simulink model "control_system_2022b"  (R2022b)
settings: Solver=VariableStepAuto  StartTime=0.0  StopTime=10.0  RelTol=1e-3
model workspace (MAT data in the model file):
  b_w = Simulink.Parameter
  b_w.Value = 150
  b_w.DataType = 'auto'
  b_w.Complexity = 'real'
  b_w.Dimensions = [1 1]
  v = Simulink.Parameter
  v.Value = 1000
  v.DataType = 'auto'
  v.Complexity = 'real'
  v.Dimensions = [1 1]
libraries: slpidlib x3
settings Model: Creator=gabrielle  LastModifiedBy=22546723@sun.ac.za
settings OptimizationCC: ReuseModelBlockBuffer=on

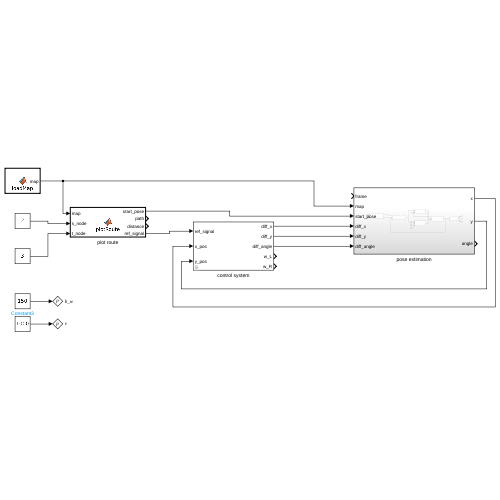
[thumbnail: Simulink's stored preview of the top-level diagram]
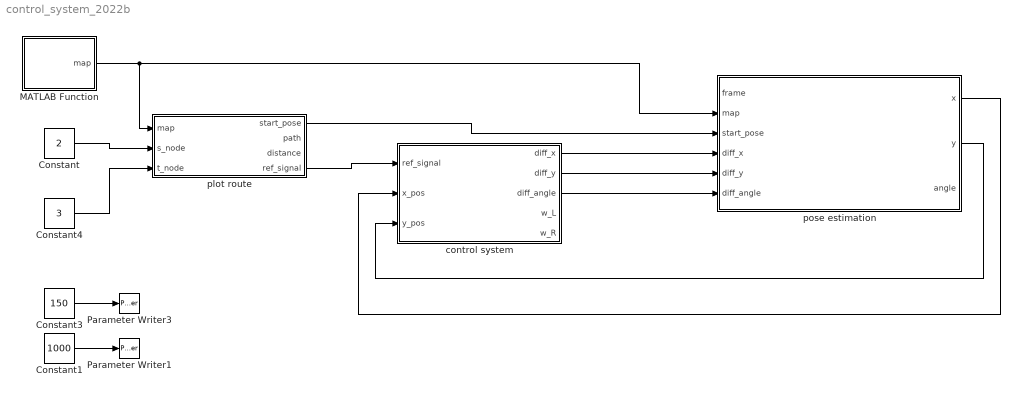
== system control_system_2022b ==
  Constant : Constant  Value=2
  Constant1 : Constant  Value=1000
  Constant3 : Constant  Value=150
  Constant4 : Constant  Value=3
  MATLAB Function : MATLAB Function  TreatAsAtomicUnit=on
  Parameter Writer1 : ParameterWriter  AccessWorkspaceVariable=on  WorkspaceVariableName=v
  Parameter Writer3 : ParameterWriter  AccessWorkspaceVariable=on  WorkspaceVariableName=b_w
  control system : Subsystem  mask{b_w=b_w, V=v}
      mask prompts: b_w "Distance between drive whels (mm)"; V "Base wheel speed (mm/s)"
  plot route : MATLAB Function  TreatAsAtomicUnit=on
  pose estimation : Subsystem
  wires:
  Constant3/1 -> Parameter Writer3/1
  Constant1/1 -> Parameter Writer1/1
  plot route/4(ref_signal) -> control system/1(ref_signal)
  control system/1(diff_x) -> pose estimation/4(diff_x)
  control system/2(diff_y) -> pose estimation/5(diff_y)
  control system/3(diff_angle) -> pose estimation/6(diff_angle)
  pose estimation/1(x) -> control system/2(x_pos)
  pose estimation/2(y) -> control system/3(y_pos)
  MATLAB Function/1(map) -> plot route/1(map), pose estimation/2(map)
  Constant/1 -> plot route/2(s_node)
  Constant4/1 -> plot route/3(t_node)
  plot route/1(start_pose) -> pose estimation/3(start_pose)

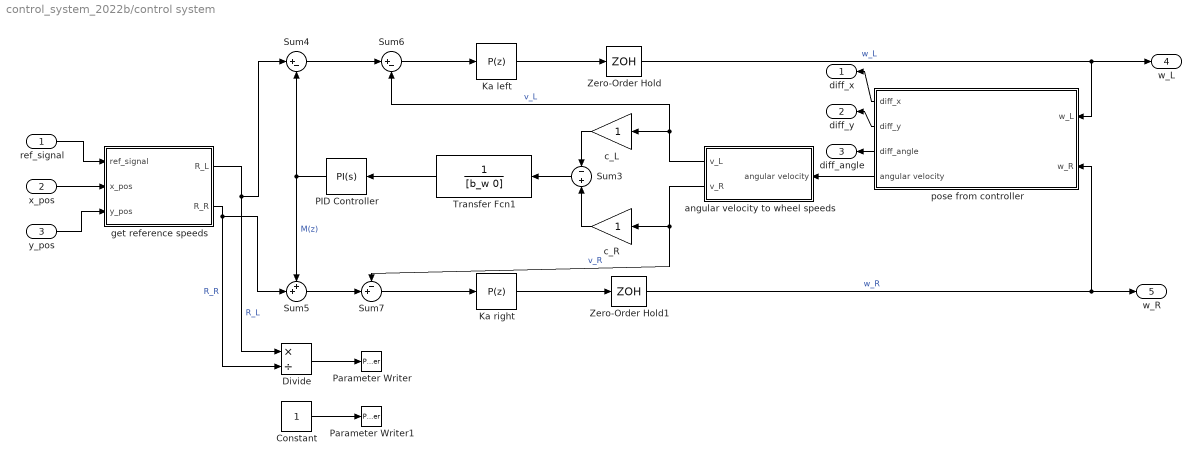
== system control_system_2022b/control system ==
  ref_signal : Inport
  x_pos : Inport  Port=2
  y_pos : Inport  Port=3
  Constant : Constant
  Divide : Product  Inputs=*/
  Ka left : slpidlib/PID Controller  Controller=P  Form=Parallel  TimeDomain=Discrete-time  UseExternalTs=off  SampleTime=-1  IntegratorMethod=Forward Euler  FilterMethod=Forward Euler  ControllerParametersSource=internal  P=1  I=1  UseKiTs=off  D=0  N=100  UseFilter=on  TunerSelectOption=Transfer Function Based (PID Tuner App)  InitialConditionSource=internal  InitialConditionForIntegrator=0  InitialConditionForFilter=0  DifferentiatorICPrevScaledInput=0  ExternalReset=none  TrackingMode=off  Kt=1  LimitOutput=off  SatLimitsSource=internal  UpperSaturationLimit=inf  LowerSaturationLimit=-inf  LinearizeAsGain=off  AntiWindupMode=none  Kb=1  LimitIntegrator=off  UpperIntegratorSaturationLimit=inf  LowerIntegratorSaturationLimit=-inf  POutMin=[]  POutMax=[]  IOutMin=[]  IOutMax=[]  DOutMin=[]  DOutMax=[]  NOutMin=[]  NOutMax=[]  SumOutMin=[]  SumOutMax=[]  SaturationOutMin=[]  SaturationOutMax=[]  PParamMin=[]  PParamMax=[]  IParamMin=[]  IParamMax=[]  DParamMin=[]  DParamMax=[]  NParamMin=[]  NParamMax=[]  KbParamMin=[]  KbParamMax=[]  KtParamMin=[]  KtParamMax=[]  KbOutMin=[]  KbOutMax=[]  KtOutMin=[]  KtOutMax=[]  IntegratorOutMin=[]  IntegratorOutMax=[]  FilterOutMin=[]  FilterOutMax=[]  SumI1OutMin=[]  SumI1OutMax=[]  SumI2OutMin=[]  SumI2OutMax=[]  SumI3OutMin=[]  SumI3OutMax=[]  SumI4OutMin=[]  SumI4OutMax=[]  SumDOutMin=[]  SumDOutMax=[]  DifferentiatorOutMin=[]  DifferentiatorOutMax=[]  FilterDiffOutCoefMin=[]  FilterDiffOutCoefMax=[]  ReciprocalOutMin=[]  ReciprocalOutMax=[]  SumDenOutMin=[]  SumDenOutMax=[]  SumNumOutMin=[]  SumNumOutMax=[]  DivideOutMin=[]  DivideOutMax=[]  UdiffTsProdOutMin=[]  UdiffTsProdOutMax=[]  NTsProdOutMin=[]  NTsProdOutMax=[]  UintegralTsProdOutMin=[]  UintegralTsProdOutMax=[]  UngainTsProdOutMin=[]  UngainTsProdOutMax=[]  ClampingZeroOutDataTypeStr=Inherit: Inherit via back propagation  ClampingZeroOutMin=[]  ClampingZeroOutMax=[]  FilterDenConstantOutDataTypeStr=Inherit: Inherit via back propagation  FilterDenConstantOutMin=[]  FilterDenConstantOutMax=[]  PCopyOutDataTypeStr=Inherit: Inherit via back propagation  PCopyOutMin=[]  PCopyOutMax=[]  NCopyOutDataTypeStr=Inherit: Inherit via back propagation  NCopyOutMin=[]  NCopyOutMax=[]  IntegratorContinuousStateAttributes=''  IntegratorStateMustResolveToSignalObject=off  IntegratorRTWStateStorageClass=Auto  FilterContinuousStateAttributes=''  FilterStateMustResolveToSignalObject=off  FilterRTWStateStorageClass=Auto  ParallelPVariant=InternalParameters  IdealPVariant=Disabled  IVariant=Disabled  DVariant=Disabled  IntegratorVariant=Disabled  SatVariant=Disabled  AWVariant=Disabled  PCopyVariant=Disabled  TRVariant=Disabled  FdbkBlocksVariant=Forward  IdealPFdbkVariant=Disabled  SatFdbkVariant=Disabled  DerivativeFilterVariant=Disabled  NVariant=Disabled  NCopyVariant=Disabled_SignalSpec  FilterICVariant=Disabled  IntegratorICVariant=Disabled  ExternalResetVariant=Disabled  TRSumVariant=Passthrough  SumFdbkVariant=Disabled  SumVariant=Passthrough_P  TsampFilterVariant=InternalTs  TsampNgainVariant=Passthrough  TsampIntegralVariant=Disabled_SignalSpec  ExternalSaturationOutDataTypeStr=Inherit: Same as second input
      settings: LibrarySourceBlock=simulink/Discrete/Discrete PID Controller
  Ka right : slpidlib/PID Controller  Controller=P  Form=Parallel  TimeDomain=Discrete-time  UseExternalTs=off  SampleTime=-1  IntegratorMethod=Forward Euler  FilterMethod=Forward Euler  ControllerParametersSource=internal  P=1  I=1  UseKiTs=off  D=0  N=100  UseFilter=on  TunerSelectOption=Transfer Function Based (PID Tuner App)  InitialConditionSource=internal  InitialConditionForIntegrator=0  InitialConditionForFilter=0  DifferentiatorICPrevScaledInput=0  ExternalReset=none  TrackingMode=off  Kt=1  LimitOutput=off  SatLimitsSource=internal  UpperSaturationLimit=inf  LowerSaturationLimit=-inf  LinearizeAsGain=off  AntiWindupMode=none  Kb=1  LimitIntegrator=off  UpperIntegratorSaturationLimit=inf  LowerIntegratorSaturationLimit=-inf  POutMin=[]  POutMax=[]  IOutMin=[]  IOutMax=[]  DOutMin=[]  DOutMax=[]  NOutMin=[]  NOutMax=[]  SumOutMin=[]  SumOutMax=[]  SaturationOutMin=[]  SaturationOutMax=[]  PParamMin=[]  PParamMax=[]  IParamMin=[]  IParamMax=[]  DParamMin=[]  DParamMax=[]  NParamMin=[]  NParamMax=[]  KbParamMin=[]  KbParamMax=[]  KtParamMin=[]  KtParamMax=[]  KbOutMin=[]  KbOutMax=[]  KtOutMin=[]  KtOutMax=[]  IntegratorOutMin=[]  IntegratorOutMax=[]  FilterOutMin=[]  FilterOutMax=[]  SumI1OutMin=[]  SumI1OutMax=[]  SumI2OutMin=[]  SumI2OutMax=[]  SumI3OutMin=[]  SumI3OutMax=[]  SumI4OutMin=[]  SumI4OutMax=[]  SumDOutMin=[]  SumDOutMax=[]  DifferentiatorOutMin=[]  DifferentiatorOutMax=[]  FilterDiffOutCoefMin=[]  FilterDiffOutCoefMax=[]  ReciprocalOutMin=[]  ReciprocalOutMax=[]  SumDenOutMin=[]  SumDenOutMax=[]  SumNumOutMin=[]  SumNumOutMax=[]  DivideOutMin=[]  DivideOutMax=[]  UdiffTsProdOutMin=[]  UdiffTsProdOutMax=[]  NTsProdOutMin=[]  NTsProdOutMax=[]  UintegralTsProdOutMin=[]  UintegralTsProdOutMax=[]  UngainTsProdOutMin=[]  UngainTsProdOutMax=[]  ClampingZeroOutDataTypeStr=Inherit: Inherit via back propagation  ClampingZeroOutMin=[]  ClampingZeroOutMax=[]  FilterDenConstantOutDataTypeStr=Inherit: Inherit via back propagation  FilterDenConstantOutMin=[]  FilterDenConstantOutMax=[]  PCopyOutDataTypeStr=Inherit: Inherit via back propagation  PCopyOutMin=[]  PCopyOutMax=[]  NCopyOutDataTypeStr=Inherit: Inherit via back propagation  NCopyOutMin=[]  NCopyOutMax=[]  IntegratorContinuousStateAttributes=''  IntegratorStateMustResolveToSignalObject=off  IntegratorRTWStateStorageClass=Auto  FilterContinuousStateAttributes=''  FilterStateMustResolveToSignalObject=off  FilterRTWStateStorageClass=Auto  ParallelPVariant=InternalParameters  IdealPVariant=Disabled  IVariant=Disabled  DVariant=Disabled  IntegratorVariant=Disabled  SatVariant=Disabled  AWVariant=Disabled  PCopyVariant=Disabled  TRVariant=Disabled  FdbkBlocksVariant=Forward  IdealPFdbkVariant=Disabled  SatFdbkVariant=Disabled  DerivativeFilterVariant=Disabled  NVariant=Disabled  NCopyVariant=Disabled_SignalSpec  FilterICVariant=Disabled  IntegratorICVariant=Disabled  ExternalResetVariant=Disabled  TRSumVariant=Passthrough  SumFdbkVariant=Disabled  SumVariant=Passthrough_P  TsampFilterVariant=InternalTs  TsampNgainVariant=Passthrough  TsampIntegralVariant=Disabled_SignalSpec  ExternalSaturationOutDataTypeStr=Inherit: Same as second input
      settings: LibrarySourceBlock=simulink/Discrete/Discrete PID Controller
  PID Controller : slpidlib/PID Controller  Controller=PI  Form=Parallel  TimeDomain=Continuous-time  UseExternalTs=off  SampleTime=-1  IntegratorMethod=Forward Euler  FilterMethod=Forward Euler  ControllerParametersSource=internal  P=1  I=1  UseKiTs=off  D=0  N=100  UseFilter=on  TunerSelectOption=Transfer Function Based (PID Tuner App)  InitialConditionSource=internal  InitialConditionForIntegrator=0  InitialConditionForFilter=0  DifferentiatorICPrevScaledInput=0  ExternalReset=none  TrackingMode=off  Kt=1  LimitOutput=off  SatLimitsSource=internal  UpperSaturationLimit=inf  LowerSaturationLimit=-inf  LinearizeAsGain=on  AntiWindupMode=none  Kb=1  LimitIntegrator=off  UpperIntegratorSaturationLimit=inf  LowerIntegratorSaturationLimit=-inf  POutMin=[]  POutMax=[]  IOutMin=[]  IOutMax=[]  DOutMin=[]  DOutMax=[]  NOutMin=[]  NOutMax=[]  SumOutMin=[]  SumOutMax=[]  SaturationOutMin=[]  SaturationOutMax=[]  PParamMin=[]  PParamMax=[]  IParamMin=[]  IParamMax=[]  DParamMin=[]  DParamMax=[]  NParamMin=[]  NParamMax=[]  KbParamMin=[]  KbParamMax=[]  KtParamMin=[]  KtParamMax=[]  KbOutMin=[]  KbOutMax=[]  KtOutMin=[]  KtOutMax=[]  IntegratorOutMin=[]  IntegratorOutMax=[]  FilterOutMin=[]  FilterOutMax=[]  SumI1OutMin=[]  SumI1OutMax=[]  SumI2OutMin=[]  SumI2OutMax=[]  SumI3OutMin=[]  SumI3OutMax=[]  SumI4OutMin=[]  SumI4OutMax=[]  SumDOutMin=[]  SumDOutMax=[]  DifferentiatorOutMin=[]  DifferentiatorOutMax=[]  FilterDiffOutCoefMin=[]  FilterDiffOutCoefMax=[]  ReciprocalOutMin=[]  ReciprocalOutMax=[]  SumDenOutMin=[]  SumDenOutMax=[]  SumNumOutMin=[]  SumNumOutMax=[]  DivideOutMin=[]  DivideOutMax=[]  UdiffTsProdOutMin=[]  UdiffTsProdOutMax=[]  NTsProdOutMin=[]  NTsProdOutMax=[]  UintegralTsProdOutMin=[]  UintegralTsProdOutMax=[]  UngainTsProdOutMin=[]  UngainTsProdOutMax=[]  ClampingZeroOutDataTypeStr=Inherit: Inherit via back propagation  ClampingZeroOutMin=[]  ClampingZeroOutMax=[]  FilterDenConstantOutDataTypeStr=Inherit: Inherit via back propagation  FilterDenConstantOutMin=[]  FilterDenConstantOutMax=[]  PCopyOutDataTypeStr=Inherit: Inherit via back propagation  PCopyOutMin=[]  PCopyOutMax=[]  NCopyOutDataTypeStr=Inherit: Inherit via back propagation  NCopyOutMin=[]  NCopyOutMax=[]  IntegratorContinuousStateAttributes=''  IntegratorStateMustResolveToSignalObject=off  IntegratorRTWStateStorageClass=Auto  FilterContinuousStateAttributes=''  FilterStateMustResolveToSignalObject=off  FilterRTWStateStorageClass=Auto  ParallelPVariant=InternalParameters  IdealPVariant=Disabled  IVariant=InternalParameters  DVariant=Disabled  IntegratorVariant=Continuous  SatVariant=Disabled  AWVariant=Passthrough  PCopyVariant=Disabled  TRVariant=Disabled  FdbkBlocksVariant=Forward  IdealPFdbkVariant=Disabled  SatFdbkVariant=Disabled  DerivativeFilterVariant=Disabled  NVariant=Disabled  NCopyVariant=Disabled_SignalSpec  FilterICVariant=Disabled  IntegratorICVariant=InternalICs  ExternalResetVariant=Disabled  TRSumVariant=Passthrough  SumFdbkVariant=Disabled  SumVariant=Sum_PI  TsampFilterVariant=InternalTs  TsampNgainVariant=Passthrough  TsampIntegralVariant=Passthrough  ExternalSaturationOutDataTypeStr=Inherit: Same as second input
  Parameter Writer : ParameterWriter  ParameterOwnerBlock=../c_R  ParameterName=Gain  ParameterInternalName=Gain
  Parameter Writer1 : ParameterWriter  ParameterOwnerBlock=../c_L  ParameterName=Gain  ParameterInternalName=Gain
  Sum3 : Sum  Inputs=-|+
  Sum4 : Sum  Inputs=|+-
  Sum5 : Sum  Inputs=++|
  Sum6 : Sum  Inputs=|+-
  Sum7 : Sum  Inputs=-+|
  Transfer Fcn1 : TransferFcn  Denominator=[b_w 0]
  Zero-Order Hold : ZeroOrderHold  SampleTime=-1
  Zero-Order Hold1 : ZeroOrderHold  SampleTime=-1
  angular velocity to wheel speeds : Subsystem
  c_L : Gain
  c_R : Gain
  get reference speeds : Subsystem
  pose from controller : Subsystem
  diff_x : Outport
  diff_y : Outport  Port=2
  diff_angle : Outport  Port=3
  w_L : Outport  Port=4
  w_R : Outport  Port=5
  wires:
  pose from controller/1(diff_x) -> diff_x/1
  Zero-Order Hold1/1 -> w_R/1, pose from controller/2(w_R)  "w_R"
  get reference speeds/1(R_L) -> Divide/1, Sum4/1  "R_L"
  pose from controller/4(angular velocity) -> angular velocity to wheel speeds/1(angular velocity)
  Sum5/1 -> Sum7/2
  Sum4/1 -> Sum6/1
  angular velocity to wheel speeds/2(v_R) -> Sum7/1, c_R/1  "v_R"
  get reference speeds/2(R_R) -> Sum5/2, Divide/2  "R_R"
  Zero-Order Hold/1 -> w_L/1, pose from controller/1(w_L)  "w_L"
  x_pos/1 -> get reference speeds/2(x_pos)
  Divide/1 -> Parameter Writer/1
  angular velocity to wheel speeds/1(v_L) -> Sum6/2, c_L/1  "v_L"
  ref_signal/1 -> get reference speeds/1(ref_signal)
  pose from controller/3(diff_angle) -> diff_angle/1
  PID Controller/1 -> Sum5/1, Sum4/2  "M(z)"
  Ka right/1 -> Zero-Order Hold1/1
  Sum6/1 -> Ka left/1
  y_pos/1 -> get reference speeds/3(y_pos)
  Sum7/1 -> Ka right/1
  Transfer Fcn1/1 -> PID Controller/1
  Ka left/1 -> Zero-Order Hold/1
  c_L/1 -> Sum3/1
  Sum3/1 -> Transfer Fcn1/1
  pose from controller/2(diff_y) -> diff_y/1
  c_R/1 -> Sum3/2
  Constant/1 -> Parameter Writer1/1

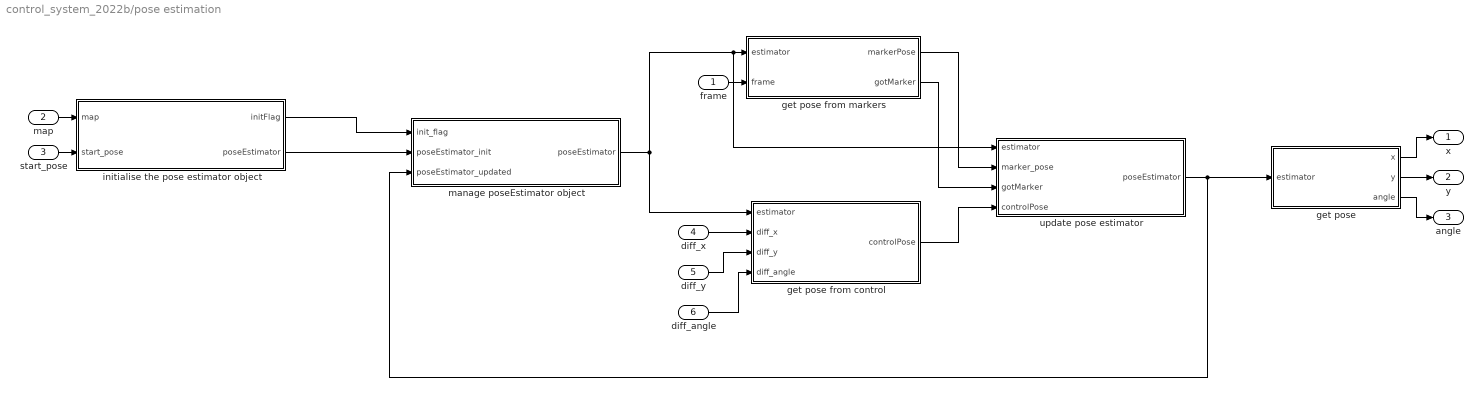
== system control_system_2022b/pose estimation ==
  frame : Inport
  map : Inport  Port=2
  start_pose : Inport  Port=3
  diff_x : Inport  Port=4
  diff_y : Inport  Port=5
  diff_angle : Inport  Port=6
  get pose : MATLAB Function  TreatAsAtomicUnit=on
  get pose from control : MATLAB Function  TreatAsAtomicUnit=on
  get pose from markers : MATLAB Function  TreatAsAtomicUnit=on
  initialise the pose estimator object : MATLAB Function  TreatAsAtomicUnit=on
  manage poseEstimator object : Subsystem
  update pose estimator : MATLAB Function  TreatAsAtomicUnit=on
  x : Outport
  y : Outport  Port=2
  angle : Outport  Port=3
  wires:
  get pose from control/1(controlPose) -> update pose estimator/4(controlPose)
  frame/1 -> get pose from markers/2(frame)
  get pose/3(angle) -> angle/1
  get pose from markers/2(gotMarker) -> update pose estimator/3(gotMarker)
  update pose estimator/1(poseEstimator) -> get pose/1(estimator), manage poseEstimator object/3(poseEstimator_updated)
  map/1 -> initialise the pose estimator object/1(map)
  manage poseEstimator object/1(poseEstimator) -> update pose estimator/1(estimator), get pose from markers/1(estimator), get pose from control/1(estimator)
  start_pose/1 -> initialise the pose estimator object/2(start_pose)
  get pose/2(y) -> y/1
  initialise the pose estimator object/1(initFlag) -> manage poseEstimator object/1(init_flag)
  diff_angle/1 -> get pose from control/4(diff_angle)
  diff_x/1 -> get pose from control/2(diff_x)
  diff_y/1 -> get pose from control/3(diff_y)
  initialise the pose estimator object/2(poseEstimator) -> manage poseEstimator object/2(poseEstimator_init)
  get pose/1(x) -> x/1
  get pose from markers/1(markerPose) -> update pose estimator/2(marker_pose)

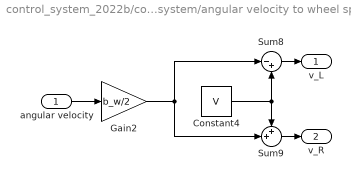
== system control_system_2022b/control system/angular velocity to wheel speeds ==
  angular velocity : Inport
  Constant4 : Constant  Value=V  VectorParams1D=off
  Gain2 : Gain  Gain=b_w/2
  Sum8 : Sum  Inputs=|-+
  Sum9 : Sum  Inputs=++|
  v_L : Outport
  v_R : Outport  Port=2
  wires:
  Sum9/1 -> v_R/1
  angular velocity/1 -> Gain2/1
  Sum8/1 -> v_L/1
  Gain2/1 -> Sum9/2, Sum8/1
  Constant4/1 -> Sum9/1, Sum8/2

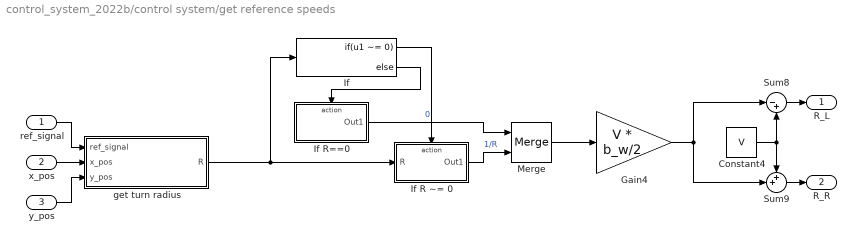
== system control_system_2022b/control system/get reference speeds ==
  ref_signal : Inport
  x_pos : Inport  Port=2
  y_pos : Inport  Port=3
  Constant4 : Constant  Value=V
  Gain4 : Gain  Gain=V * b_w/2
  If : If  IfExpression=u1 ~= 0
  If R ~= 0 : Subsystem  TreatAsAtomicUnit=on
  If R==0 : Subsystem  TreatAsAtomicUnit=on
  Merge : Merge  InitialOutput=0
  Sum8 : Sum  Inputs=|-+
  Sum9 : Sum  Inputs=++|
  get turn radius : MATLAB Function  TreatAsAtomicUnit=on
  R_L : Outport
  R_R : Outport  Port=2
  wires:
  x_pos/1 -> get turn radius/2(x_pos)
  y_pos/1 -> get turn radius/3(y_pos)
  Merge/1 -> Gain4/1
  Sum9/1 -> R_R/1
  Gain4/1 -> Sum8/1, Sum9/2
  If/1 -> If R ~= 0/Action
  If/2 -> If R==0/Action
  If R==0/1(Out1) -> Merge/1  "0"
  Constant4/1 -> Sum9/1, Sum8/2
  If R ~= 0/1(Out1) -> Merge/2  "1/R"
  Sum8/1 -> R_L/1
  get turn radius/1(R) -> If/1, If R ~= 0/1(R)
  ref_signal/1 -> get turn radius/1(ref_signal)

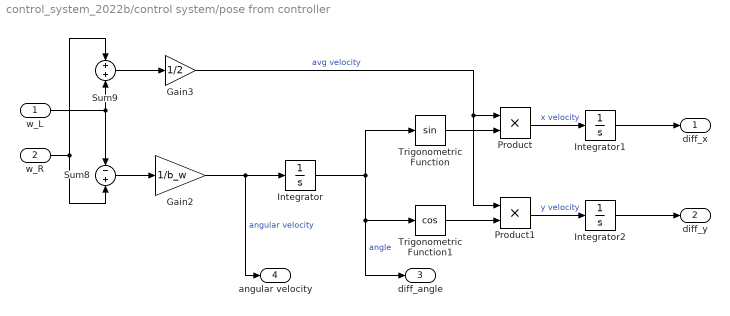
== system control_system_2022b/control system/pose from controller ==
  w_L : Inport
  w_R : Inport  Port=2
  Gain2 : Gain  Gain=1/b_w
  Gain3 : Gain  Gain=1/2
  Integrator : Integrator
  Integrator1 : Integrator
  Integrator2 : Integrator
  Product : Product
  Product1 : Product
  Sum8 : Sum  Inputs=-|+
  Sum9 : Sum  Inputs=+|+
  Trigonometric Function : Trigonometry
  Trigonometric Function1 : Trigonometry  Operator=cos
  diff_x : Outport
  diff_y : Outport  Port=2
  diff_angle : Outport  Port=3
  angular velocity : Outport  Port=4
  wires:
  Integrator2/1 -> diff_y/1
  Product/1 -> Integrator1/1  "x velocity"
  Sum9/1 -> Gain3/1
  Integrator1/1 -> diff_x/1
  Product1/1 -> Integrator2/1  "y velocity"
  w_R/1 -> Sum8/2, Sum9/1
  Trigonometric Function1/1 -> Product1/2
  Gain3/1 -> Product/1, Product1/1  "avg velocity"
  Trigonometric Function/1 -> Product/2
  Integrator/1 -> diff_angle/1, Trigonometric Function1/1, Trigonometric Function/1  "angle"
  Gain2/1 -> angular velocity/1, Integrator/1  "angular velocity"
  w_L/1 -> Sum8/1, Sum9/2
  Sum8/1 -> Gain2/1

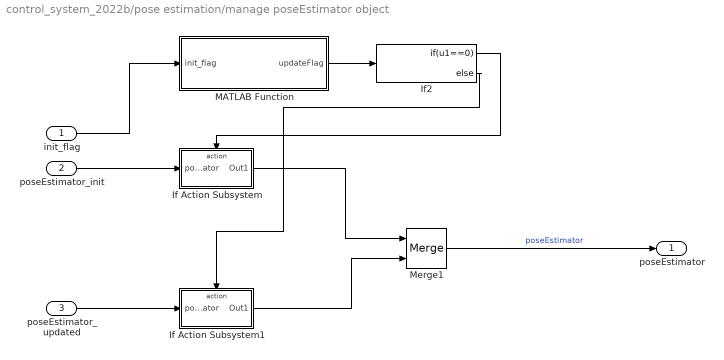
== system control_system_2022b/pose estimation/manage poseEstimator object ==
  init_flag : Inport
  poseEstimator_init : Inport  Port=2
  poseEstimator_updated : Inport  Port=3
  If Action Subsystem : Subsystem  TreatAsAtomicUnit=on
  If Action Subsystem1 : Subsystem  TreatAsAtomicUnit=on
  If2 : If  IfExpression=u1==0
  MATLAB Function : MATLAB Function  TreatAsAtomicUnit=on
  Merge1 : Merge  InitialOutput=0
  poseEstimator : Outport
  wires:
  MATLAB Function/1(updateFlag) -> If2/1
  If2/1 -> If Action Subsystem/Action
  If Action Subsystem/1(Out1) -> Merge1/1
  If Action Subsystem1/1(Out1) -> Merge1/2
  If2/2 -> If Action Subsystem1/Action
  Merge1/1 -> poseEstimator/1  "poseEstimator"
  init_flag/1 -> MATLAB Function/1(init_flag)
  poseEstimator_updated/1 -> If Action Subsystem1/1(poseEstimator)
  poseEstimator_init/1 -> If Action Subsystem/1(poseEstimator)

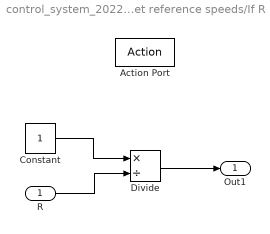
== system control_system_2022b/control system/get reference speeds/If R ~= 0 ==
  R : Inport
  Action Port : ActionPort  ActionPortLabel=if(u1 ~= 0)
  Constant : Constant
  Divide : Product  Inputs=*/
  Out1 : Outport
  wires:
  Constant/1 -> Divide/1
  R/1 -> Divide/2
  Divide/1 -> Out1/1

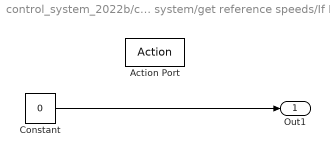
== system control_system_2022b/control system/get reference speeds/If R==0 ==
  Action Port : ActionPort  ActionPortLabel=else
  Constant : Constant  Value=0
  Out1 : Outport
  wires:
  Constant/1 -> Out1/1

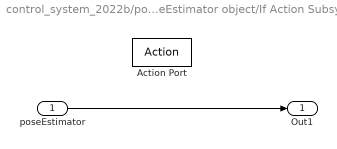
== system control_system_2022b/pose estimation/manage poseEstimator object/If Action Subsystem ==
  poseEstimator : Inport
  Action Port : ActionPort  ActionPortLabel=if(u1==0)
  Out1 : Outport
  wires:
  poseEstimator/1 -> Out1/1

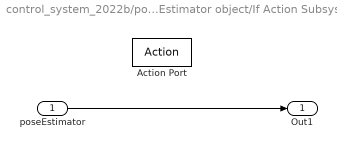
== system control_system_2022b/pose estimation/manage poseEstimator object/If Action Subsystem1 ==
  poseEstimator : Inport
  Action Port : ActionPort  ActionPortLabel=else
  Out1 : Outport
  wires:
  poseEstimator/1 -> Out1/1

== matlab function control_system_2022b/plot route ==
  data: start_pose output; path output; distance output; ref_signal output; map input; s_node input; t_node input
function [start_pose, path, distance, ref_signal] = plotRoute(map, s_node, t_node)
% plotRoute     plot the route from the start node to the stop node
% Inputs:
%   map     : current map object
%   s_node  : starting node id
%   t_node  : stop node id
% Outputs:
%   path        : shortest path between the two nodes - array of node IDs
%   distance    : total distance of path
%   ref_signal  : reference signal for the path - cell array of
%                   path_segment objects
%
% See also map, path_segment

routePlanner = route_planner(map);
[path, distance] = plot_route(routePlanner, s_node, t_node);

ref_signal = convert_to_ref(routePlanner, path);

start_pose = map.nodes{s_node};
start_pose = [start_pose.x_coord; start_pose.y_coord];

== matlab function control_system_2022b/control system/get reference speeds/get turn radius ==
  data: ref_signal input; R output; x_pos input; y_pos input
function R = getRadius(ref_signal, x_pos, y_pos)
% getRadius     get the turn radius of the current path segment
% Inputs:
%   ref_signal  : reference signal - cell array of path_segments
%   x_pos       : estimated x coordinate
%   y_pos       : estimated y coordinate
%
% Outputs:
%   R   : turn radius of current path segment
%
% See also path_segment

persistent n

if isempty(n)
    n = 1;
end

segment = ref_signal{n};
R = segment.R;

x_check = (x_pos <= segment.stop(1)*0.9) && (x_pos >= segment.stop(1)*1.1); % x_pos within 10% of stop node x coord
y_check = (y_pos <= segment.stop(2)*0.9) && (y_pos >= segment.stop(2)*1.1); % y_pos within 10% of stop node y coord

if x_check && y_check
    n = n+1;
end

== matlab function control_system_2022b/pose estimation/initialise the pose estimator object ==
  data: initFlag output; poseEstimator output; map input; start_pose input
function [initFlag, poseEstimator] = initPoseEstimator(map, start_pose)
poseEstimator = pose_estimator(map, start_pose);
initFlag = 0;

== matlab function control_system_2022b/pose estimation/get pose from markers ==
  data: estimator input; markerPose output; frame input; gotMarker output
function [markerPose, gotMarker] = getMarkerPose(estimator, frame)
if ~isempty(frame)
    [id, loc, pose] = find_markers(estimator, frame);
    markerPose = pose_from_marker(estimator, loc, pose);
    gotMarker = 1;
else
    markerPose = [404; 404; 404];
    gotMarker = 0;
end

== matlab function control_system_2022b/pose estimation/get pose from control ==
  data: controlPose output; estimator input; diff_x input; diff_y input; diff_angle input
function controlPose = getControlPose(estimator, diff_x, diff_y, diff_angle)
controlPose = pose_from_control(estimator, diff_x, diff_y, diff_angle);

== matlab function control_system_2022b/pose estimation/update pose estimator ==
  data: estimator input; poseEstimator output; marker_pose input; gotMarker input; controlPose input
function poseEstimator  = updateEstimator(estimator, marker_pose, gotMarker, controlPose)
poseEstimator = update_pose(estimator, marker_pose, gotMarker, controlPose);

== matlab function control_system_2022b/pose estimation/manage poseEstimator object/MATLAB Function ==
  data: init_flag input; updateFlag output
function updateFlag = manageFlag(init_flag)
persistent flag

if (isempty(flag)&&(init_flag == 1))
    flag = 0;
elseif (flag == 0)
    flag = 1;
end

updateFlag = flag;

== matlab function control_system_2022b/pose estimation/get pose ==
  data: x output; estimator input; y output; angle output
function [x, y, angle] = getCurrentPose(estimator)
currentPose = get_current_pose(estimator);
x = currentPose(1);
y = currentPose(2);
angle = currentPose(3);

== matlab function control_system_2022b/MATLAB Function ==
  data: map output
function map = loadMap()
map =  load('Maps/path_segment_test.mat');
map = map.map_data;
